simulink model "W1P3"  (R2020b)
settings: Solver=VariableStepAuto  StartTime=0.0  StopTime=0.1  RelTol=1e-3
settings Model: Creator=saadh  LastModifiedBy=saadh

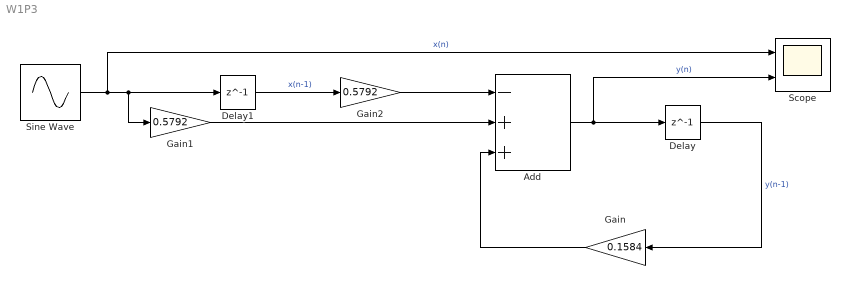
== system W1P3 ==
  Add : Sum  Inputs=-++
  Delay : Delay  DelayLength=1
  Delay1 : Delay  DelayLength=1
  Gain : Gain  Gain=0.1584
  Gain1 : Gain  Gain=0.5792
  Gain2 : Gain  Gain=0.5792
  Scope : Scope  NumInputPorts=2
  Sine Wave : Sin  Frequency=2*pi*5000  SampleTime=1/5000
  wires:
  Add/1 -> Scope/2, Delay/1  "y(n)"
  Delay/1 -> Gain/1  "y(n-1)"
  Gain/1 -> Add/3
  Delay1/1 -> Gain2/1  "x(n-1)"
  Gain2/1 -> Add/1
  Gain1/1 -> Add/2
  Sine Wave/1 -> Scope/1, Gain1/1, Delay1/1  "x(n)"
